simulink model "Lotkasim"  (R2024b)
settings: Solver=VariableStepAuto  StartTime=0.0  StopTime=30  RelTol=1e-3
values from neighbouring files (symbols this model uses):
  a = 0.6    [Lotka.m]    (also in MocGrzalkiPI.m = 2; PrawyCz1.m = 2; PrawyCz2.m = 2; Spr2.m = 2)
  b = 0.5    [Lotka.m]
  P = 10    [Lotka.m]
  Rp = 0.8    [Lotka.m]
  Rv = 1.2    [Lotka.m]
  V = 20    [Lotka.m]
settings Model: Creator=pawli  LastModifiedBy=pawli

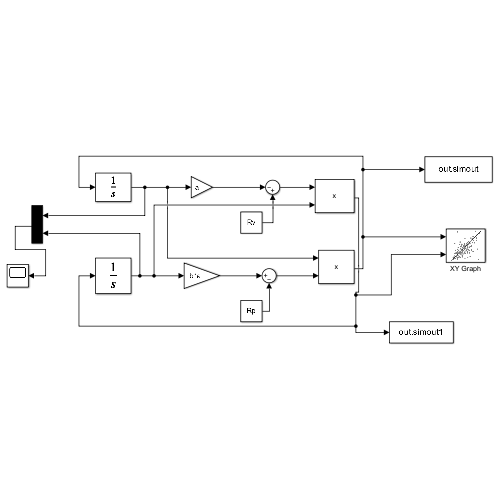
[thumbnail: Simulink's stored preview of the top-level diagram]
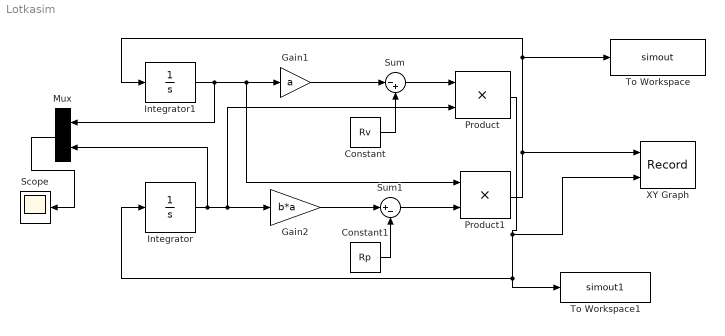
== system Lotkasim ==
  Constant : Constant  Value=Rv
  Constant1 : Constant  Value=Rp
  Gain1 : Gain  Gain=a
  Gain2 : Gain  Gain=b*a
  Integrator : Integrator  InitialCondition=V
  Integrator1 : Integrator  InitialCondition=P
  Mux : Mux  Inputs=2
  Product : Product
  Product1 : Product
  Scope : Scope
  Sum : Sum  Inputs=|-+
  Sum1 : Sum  Inputs=|+-
  To Workspace : ToWorkspace  VariableName=simout  SampleTime=-1
  To Workspace1 : ToWorkspace  VariableName=simout1  SaveFormat=Timeseries  SampleTime=-1
  XY Graph : Record  FileSettingsInternal="{\"entries\":[{\"content\":{\"excelSettings\":{\"content\":{},\"type\":\"Streamout.ExcelSettings\"}},\"type\":\"Streamout.FileSettingStorage\",\"uuid\":\"\"}],\"packageUris\":[\"http:\\/\\/schema.mathworks.com\\/mf0\\/streamout_blocks\\/R2020a\"],\"version\":\"1.0\"}"  Layout=[1 1]  SignalsInternal="{\"entries\":[{\"content\":{\"signals\":[{\"content\":{\"blockPath\":[],\"dimensions\":[1],\"domain\":\"\",\"lineColor\":\"#a2142f\",\"plots\":[ 1 ],\"port\":1,\"sid\":[\"\"],\"signalID\":1,\"signalName\":\"Product1\"},\"type\":\"RecordBlkView.Signal\",\"uuid\":\"\"},{\"content\":{\"blockPath\":[],\"dimensions\":[1],\"domain\":\"\",\"lineColor\":\"#139fff\",\"plots\":[ 1 ],\"port\":2,\"sid\":[\"\"],\"signalID\":2,\"signalName\":\"Product\"},\"type\":\"RecordBlkView.Signal\",\"uuid\":\"\"}]},\"type\":\"RecordBlkView.InputSignals\",\"uuid\":\"\"}],\"packageUris\":[\"http:\\/\\/schema.mathworks.com\\/mf0\\/streamout_blocks\\/R2020a\"],\"version\":\"1.0\"}"  VisualizationBindings="{\"xyplotplugin\":{\"info\":[{\"series\":[{\"bindingParametersList\":[{\"parameter\":\"X-Axis\",\"signalID\":1,\"signalName\":\"Product1\"},{\"parameter\":\"Y-Axis\",\"signalID\":2,\"signalName\":\"Product\"}],\"seriesID\":0}],\"subplotID\":1}]}}"  CompatibilityTag=XY
  wires:
  Integrator/1 -> Mux/2, Product/2, Gain2/1
  Integrator1/1 -> Mux/1, Product1/1, Gain1/1
  Gain1/1 -> Sum/1
  Constant/1 -> Sum/2
  Constant1/1 -> Sum1/2
  Gain2/1 -> Sum1/1
  Sum1/1 -> Product1/2
  Sum/1 -> Product/1
  Product/1 -> To Workspace1/1, Integrator/1, XY Graph/2
  Product1/1 -> To Workspace/1, Integrator1/1, XY Graph/1
  Mux/1 -> Scope/1
